simulink subsystem "ApplicationAbstractionMotorSwap"  (R2024a)
settings: Solver=VariableStepAuto  StartTime=0.0  StopTime=10.0  RelTol=1e-3
values from neighbouring files (symbols this model uses):
  Ts = T_pwm    [mcbMotorSwapData.m]
undefined symbols (not defined in the file or in its folder): pmsm
libraries: mcbpositiondecoderlib x6, simulink x3, mcbcontrolslib x2
settings Model: Creator=The MathWorks, Inc.  LastModifiedBy=snarayan
settings RTWCC: GPUComputeCapability=3.5

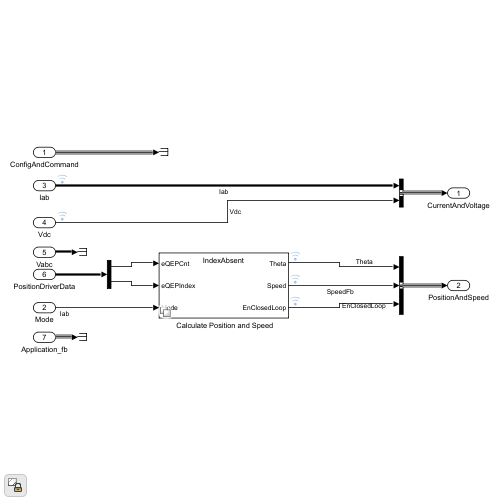
[thumbnail: Simulink's stored preview of the top-level diagram]
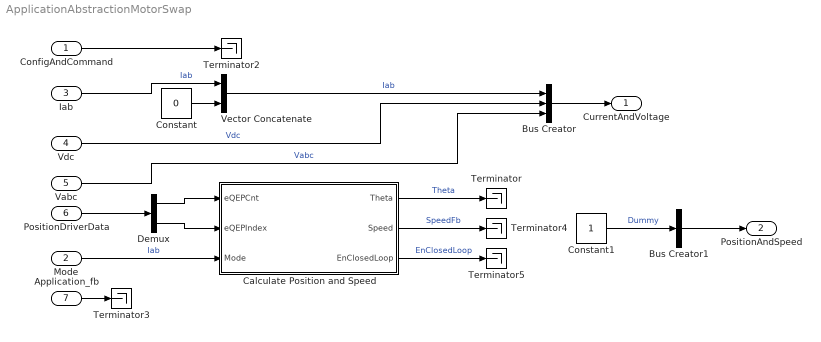
== system ApplicationAbstractionMotorSwap ==
  ConfigAndCommand : Inport
  Mode : Inport  Port=2
  Iab : Inport  Port=3
  Vdc : Inport  Port=4
  Vabc : Inport  Port=5
  PositionDriverData : Inport  Port=6
  Application_fb : Inport  Port=7
  " Calculate Position and Speed" : Subsystem  Variant=on
  Bus Creator : BusCreator  Inputs=3
  Bus Creator1 : BusCreator  Inputs=1
  Constant : Constant  Value=0  OutDataTypeStr=dataType
  Constant1 : Constant  OutDataTypeStr=dataType  SampleTime=Ts
  Demux : Demux  Outputs=2
  Terminator{,2..5} (5 alike) : Terminator
  Vector Concatenate : Concatenate
  CurrentAndVoltage : Outport
  PositionAndSpeed : Outport  Port=2
  wires:
  Vdc/1 -> Bus Creator/2  "Vdc"
  PositionDriverData/1 -> Demux/1
  Bus Creator/1 -> CurrentAndVoltage/1
  Vector Concatenate/1 -> Bus Creator/1  "Iab"
  ConfigAndCommand/1 -> Terminator2/1
  Demux/1 -> " Calculate Position and Speed"/1(eQEPCnt)
  Demux/2 -> " Calculate Position and Speed"/2(eQEPIndex)
  Mode/1 -> " Calculate Position and Speed"/3(Mode)  "Iab"
  Application_fb/1 -> Terminator3/1
  Iab/1 -> Vector Concatenate/1  "Iab"
  Constant/1 -> Vector Concatenate/2
  " Calculate Position and Speed"/1(Theta) -> Terminator/1  "Theta"
  " Calculate Position and Speed"/2(Speed) -> Terminator4/1  "SpeedFb"
  " Calculate Position and Speed"/3(EnClosedLoop) -> Terminator5/1  "EnClosedLoop"
  Bus Creator1/1 -> PositionAndSpeed/1
  Constant1/1 -> Bus Creator1/1  "Dummy"
  Vabc/1 -> Bus Creator/3  "Vabc"

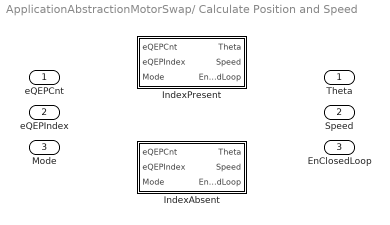
== system ApplicationAbstractionMotorSwap/ Calculate Position and Speed ==
  eQEPCnt : Inport
  eQEPIndex : Inport  Port=2
  Mode : Inport  Port=3
  IndexAbsent : Subsystem  VariantControl=pmsm.QEPIndexPresent == false
  IndexPresent : Subsystem  VariantControl=pmsm.QEPIndexPresent == true
  Theta : Outport
  Speed : Outport  Port=2
  EnClosedLoop : Outport  Port=3

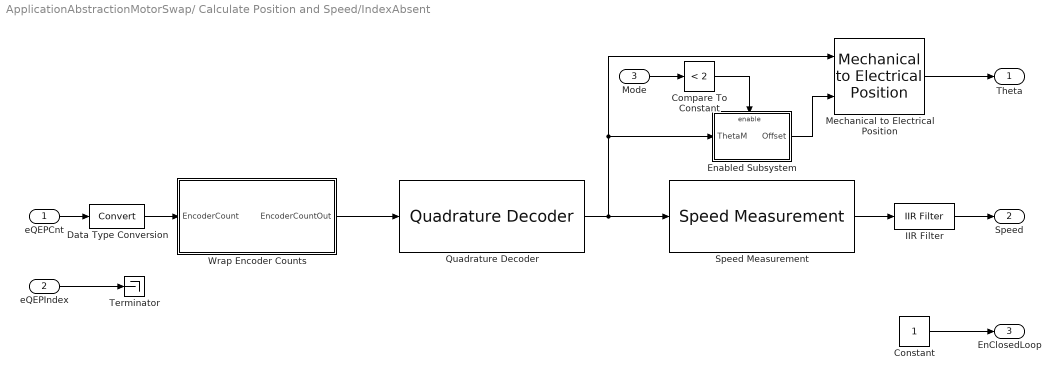
== system ApplicationAbstractionMotorSwap/ Calculate Position and Speed/IndexAbsent ==
  eQEPCnt : Inport
  eQEPIndex : Inport  Port=2
  Mode : Inport  Port=3
  Compare To Constant : simulink/Logic and Bit Operations/Compare To Constant  relop=<  const=2  OutDataTypeStr=boolean
  Constant : Constant  OutDataTypeStr=dataType
  Data Type Conversion : DataTypeConversion  RndMeth=Simplest  SaturateOnIntegerOverflow=off
  Enabled Subsystem : Subsystem  TreatAsAtomicUnit=on
  IIR Filter : mcbcontrolslib/IIR Filter  VariantControl=Low Pass Filter  VariantSelect=Low-pass  FilterConstantInputType=Specify via dialog  Filter_constant=0.01  advancedSettings=off  Ts=50e-6  cutOff_freq=32.1525
  Mechanical to Electrical Position : mcbpositiondecoderlib/Mechanical to Electrical Position  PolePairsInputType=Specify via dialog  NrPP=pmsm.p  selectedRange=Radians  MechOfstInputType=Input port  mechOffsetIn=0  maxAngleIn=2*pi  InputDataType=dataType  VariantSelect=floating-point
  Quadrature Decoder : mcbpositiondecoderlib/Quadrature Decoder  EncoderSlitsPerRevolution=pmsm.QEPSlits  EncoderCountsPerSlit=4  CounterSize=16 bits  ExternalIndexCount=off  PositionUnit=Radians  PositionDataType=dataType  ParameterInputType=off  CountsPerRevInverseDataType=single
  Speed Measurement : mcbpositiondecoderlib/Speed Measurement  PositionUnit=Radians  PositionScalingDatatype=uint32  SpeedCalculationMode=Time interval for speed calculation  SampleTimeAsync=Ts  MaximumApplicationSpeed=6000  SpeedResolution=5e-6  DelayLength=20  MaximumMeasurableSpeed=23999  MeasurableSpeedResolution=1.1176e-05  SpeedUnit=Radians/Sec  PerUnitSpeed=PU_System.N_base  SpeedDataType=dataType
  Terminator : Terminator
  Wrap Encoder Counts : Subsystem  mask{EnCountPerRev=pmsm.QEPSlits*4}
      mask prompts: EnCountPerRev "Encoder counts per rev"
  Theta : Outport
  Speed : Outport  Port=2
  EnClosedLoop : Outport  Port=3
  wires:
  Enabled Subsystem/1(Offset) -> Mechanical to Electrical Position/2
  Wrap Encoder Counts/1(EncoderCountOut) -> Quadrature Decoder/1
  Data Type Conversion/1 -> Wrap Encoder Counts/1(EncoderCount)
  Compare To Constant/1 -> Enabled Subsystem/Enable
  Mode/1 -> Compare To Constant/1
  Constant/1 -> EnClosedLoop/1
  IIR Filter/1 -> Speed/1
  Mechanical to Electrical Position/1 -> Theta/1
  eQEPIndex/1 -> Terminator/1
  Speed Measurement/1 -> IIR Filter/1
  eQEPCnt/1 -> Data Type Conversion/1
  Quadrature Decoder/1 -> Enabled Subsystem/1(ThetaM), Mechanical to Electrical Position/1, Speed Measurement/1

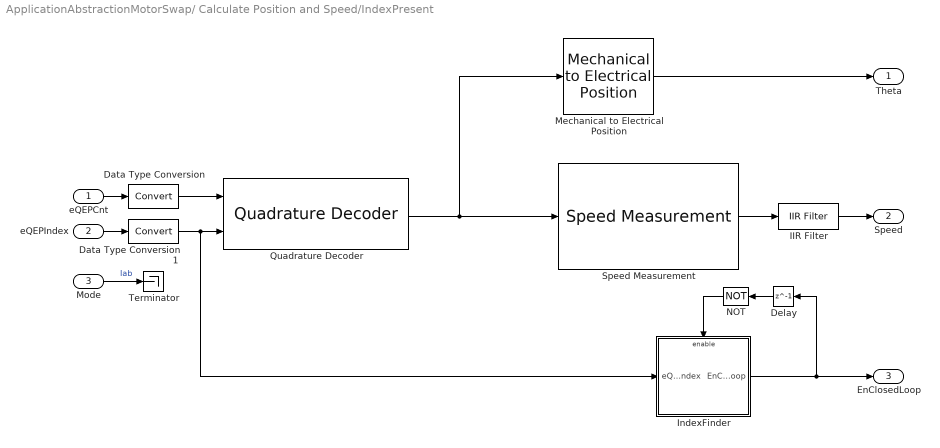
== system ApplicationAbstractionMotorSwap/ Calculate Position and Speed/IndexPresent ==
  eQEPCnt : Inport
  eQEPIndex : Inport  Port=2
  Mode : Inport  Port=3
  Data Type Conversion : DataTypeConversion  RndMeth=Simplest  SaturateOnIntegerOverflow=off
  Data Type Conversion1 : DataTypeConversion  RndMeth=Simplest  SaturateOnIntegerOverflow=off
  Delay : Delay  DelayLength=1
  IIR Filter : mcbcontrolslib/IIR Filter  VariantControl=Low Pass Filter  VariantSelect=Low-pass  FilterConstantInputType=Specify via dialog  Filter_constant=0.01  advancedSettings=off  Ts=50e-6  cutOff_freq=32.1525
  IndexFinder : Subsystem
  Mechanical to Electrical Position : mcbpositiondecoderlib/Mechanical to Electrical Position  PolePairsInputType=Specify via dialog  NrPP=pmsm.p  selectedRange=Radians  MechOfstInputType=Specify via dialog  mechOffsetIn=pmsm.PositionOffset  maxAngleIn=2*pi  InputDataType=dataType  VariantSelect=floating-point
  NOT : Logic  Operator=NOT  AllPortsSameDT=off  OutDataTypeStr=boolean
  Quadrature Decoder : mcbpositiondecoderlib/Quadrature Decoder  EncoderSlitsPerRevolution=pmsm.QEPSlits  EncoderCountsPerSlit=4  CounterSize=16 bits  ExternalIndexCount=on  PositionUnit=Radians  PositionDataType=dataType  ParameterInputType=off  CountsPerRevInverseDataType=single
  Speed Measurement : mcbpositiondecoderlib/Speed Measurement  PositionUnit=Radians  PositionScalingDatatype=uint32  SpeedCalculationMode=Time interval for speed calculation  SampleTimeAsync=Ts  MaximumApplicationSpeed=6000  SpeedResolution=5e-6  DelayLength=20  MaximumMeasurableSpeed=-0.98352  MeasurableSpeedResolution=7.6757e-12  SpeedUnit=Radians/Sec  PerUnitSpeed=PU_System.N_base  SpeedDataType=dataType
  Terminator : Terminator
  Theta : Outport
  Speed : Outport  Port=2
  EnClosedLoop : Outport  Port=3
  wires:
  Data Type Conversion1/1 -> Quadrature Decoder/2, IndexFinder/1(eQEPIndex)
  Data Type Conversion/1 -> Quadrature Decoder/1
  Delay/1 -> NOT/1
  NOT/1 -> IndexFinder/Enable
  eQEPIndex/1 -> Data Type Conversion1/1
  IndexFinder/1(EnClosedLoop) -> Delay/1, EnClosedLoop/1
  Mode/1 -> Terminator/1  "Iab"
  IIR Filter/1 -> Speed/1
  Speed Measurement/1 -> IIR Filter/1
  eQEPCnt/1 -> Data Type Conversion/1
  Mechanical to Electrical Position/1 -> Theta/1
  Quadrature Decoder/1 -> Mechanical to Electrical Position/1, Speed Measurement/1

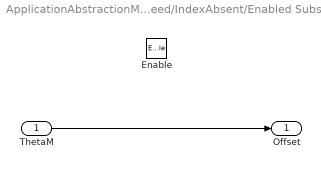
== system ApplicationAbstractionMotorSwap/ Calculate Position and Speed/IndexAbsent/Enabled Subsystem ==
  ThetaM : Inport
  Enable : EnablePort
  Offset : Outport
  wires:
  ThetaM/1 -> Offset/1

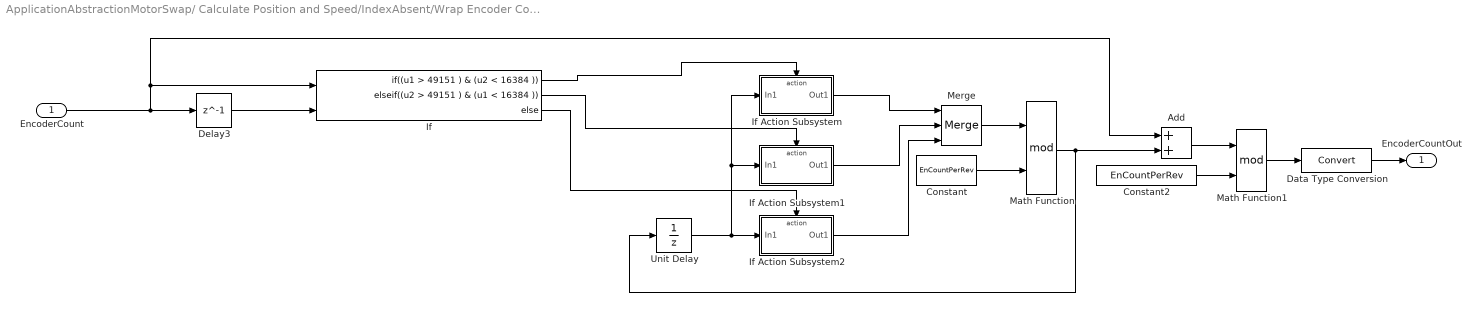
== system ApplicationAbstractionMotorSwap/ Calculate Position and Speed/IndexAbsent/Wrap Encoder Counts ==
  EncoderCount : Inport
  Add : Sum  OutDataTypeStr=single
  Constant : Constant  Value=EnCountPerRev  OutDataTypeStr=Inherit: Inherit via back propagation
  Constant2 : Constant  Value=EnCountPerRev  OutDataTypeStr=Inherit: Inherit via back propagation
  Data Type Conversion : DataTypeConversion  RndMeth=Simplest  SaturateOnIntegerOverflow=off
  Delay3 : Delay  DelayLength=1  InitialCondition=0
  If : If  NumInputs=2  IfExpression=(u1 > 49151 ) & (u2 < 16384 )  ElseIfExpressions=(u2 > 49151 ) & (u1 < 16384 )
  If Action Subsystem : Subsystem  TreatAsAtomicUnit=on
  If Action Subsystem1 : Subsystem  TreatAsAtomicUnit=on
  If Action Subsystem2 : Subsystem  TreatAsAtomicUnit=on
  Math Function : Math  Operator=mod  SignedPower=on
  Math Function1 : Math  Operator=mod  SignedPower=on
  Merge : Merge  Inputs=3
  Unit Delay : UnitDelay  SampleTime=-1  HasFrameUpgradeWarning=on
  EncoderCountOut : Outport
  wires:
  EncoderCount/1 -> Add/1, If/1, Delay3/1
  If Action Subsystem2/1(Out1) -> Merge/3
  If/2 -> If Action Subsystem1/Action
  If Action Subsystem1/1(Out1) -> Merge/2
  Unit Delay/1 -> If Action Subsystem/1(In1), If Action Subsystem1/1(In1), If Action Subsystem2/1(In1)
  If/3 -> If Action Subsystem2/Action
  If Action Subsystem/1(Out1) -> Merge/1
  Constant/1 -> Math Function/2
  Delay3/1 -> If/2
  Merge/1 -> Math Function/1
  If/1 -> If Action Subsystem/Action
  Math Function/1 -> Unit Delay/1, Add/2
  Add/1 -> Math Function1/1
  Constant2/1 -> Math Function1/2
  Math Function1/1 -> Data Type Conversion/1
  Data Type Conversion/1 -> EncoderCountOut/1

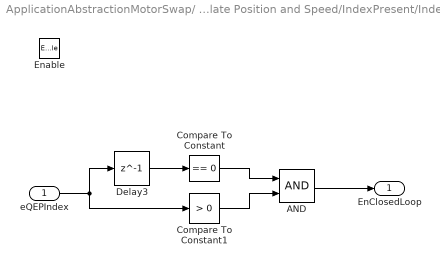
== system ApplicationAbstractionMotorSwap/ Calculate Position and Speed/IndexPresent/IndexFinder ==
  eQEPIndex : Inport
  Enable : EnablePort
  AND : Logic  AllPortsSameDT=off  OutDataTypeStr=boolean
  Compare To Constant : simulink/Logic and Bit Operations/Compare To Constant  relop===  const=0  OutDataTypeStr=boolean
  Compare To Constant1 : simulink/Logic and Bit Operations/Compare To Constant  relop=>  const=0  OutDataTypeStr=boolean
  Delay3 : Delay  DelayLength=1
  EnClosedLoop : Outport
  wires:
  AND/1 -> EnClosedLoop/1
  Delay3/1 -> Compare To Constant/1
  Compare To Constant/1 -> AND/1
  Compare To Constant1/1 -> AND/2
  eQEPIndex/1 -> Compare To Constant1/1, Delay3/1

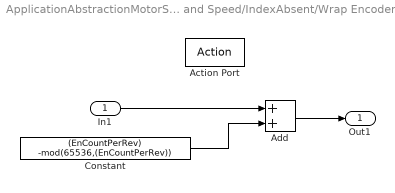
== system ApplicationAbstractionMotorSwap/ Calculate Position and Speed/IndexAbsent/Wrap Encoder Counts/If Action Subsystem ==
  In1 : Inport
  Action Port : ActionPort
  Add : Sum
  Constant : Constant  Value=(EnCountPerRev) -mod(65536,(EnCountPerRev))  OutDataTypeStr=uint16
  Out1 : Outport
  wires:
  In1/1 -> Add/1
  Constant/1 -> Add/2
  Add/1 -> Out1/1

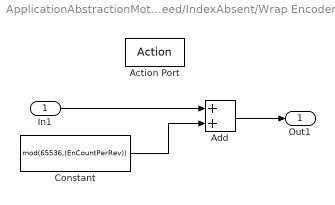
== system ApplicationAbstractionMotorSwap/ Calculate Position and Speed/IndexAbsent/Wrap Encoder Counts/If Action Subsystem1 ==
  In1 : Inport
  Action Port : ActionPort
  Add : Sum
  Constant : Constant  Value=mod(65536,(EnCountPerRev))  OutDataTypeStr=uint16
  Out1 : Outport
  wires:
  Add/1 -> Out1/1
  Constant/1 -> Add/2
  In1/1 -> Add/1

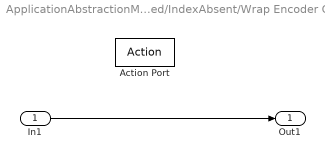
== system ApplicationAbstractionMotorSwap/ Calculate Position and Speed/IndexAbsent/Wrap Encoder Counts/If Action Subsystem2 ==
  In1 : Inport
  Action Port : ActionPort
  Out1 : Outport
  wires:
  In1/1 -> Out1/1
